simulink model "sat_sim_open_loop"  (R2022b)
settings: Solver=FixedStepAuto  StartTime=0.0  StopTime=10.0  FixedStep=0.01  RelTol=1e-3
values from neighbouring files (symbols this model uses):
  Isat = 0.00042853    [sat_params.m]
  Iwheel = 0.0019098    [sat_params.m]
  Km = -2.465    [sat_params.m]
  tau = 0.1    [sat_params.m]
libraries: slpidlib x2, simulink x1
settings Model: Creator=gigliaadmin  LastModifiedBy=micha
settings SolverCC: EnableFixedStepZeroCrossing=on

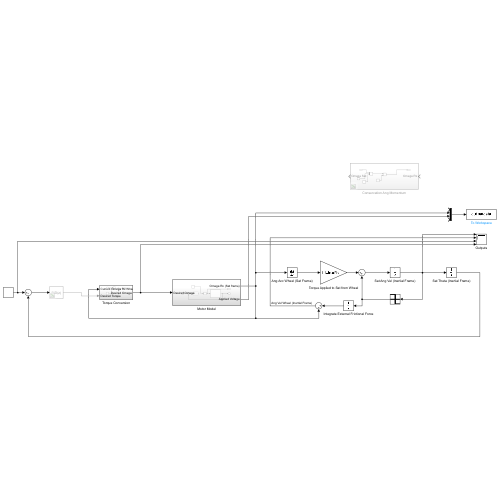
[thumbnail: Simulink's stored preview of the top-level diagram]
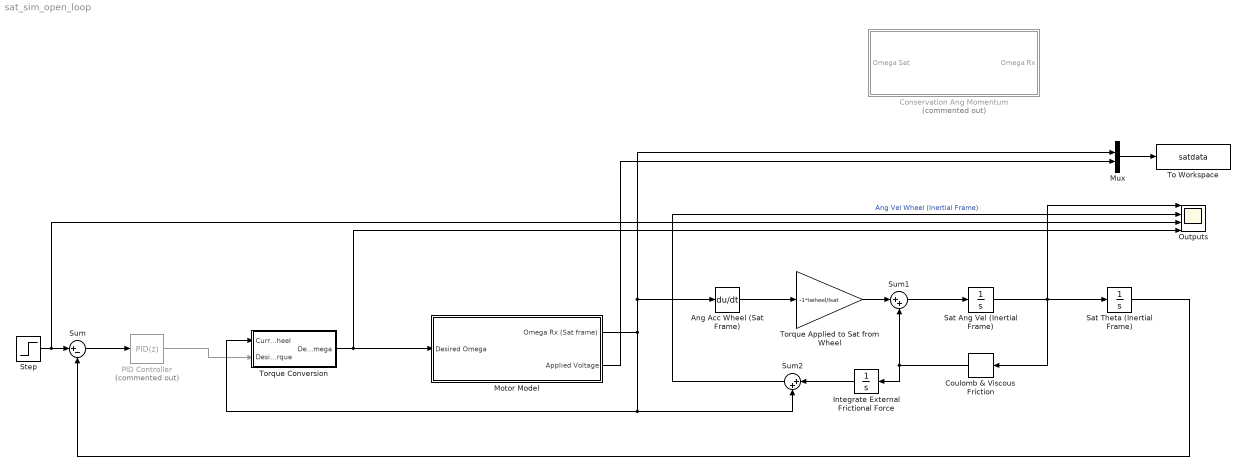
== system sat_sim_open_loop ==
  Ang Acc Wheel (Sat Frame) : Derivative
  Conservation Ang Momentum : Subsystem  Commented=on
  Coulomb & Viscous Friction : simulink/Discontinuities/Coulomb & Viscous Friction  offset=-400  gain=0
  Integrate External Frictional Force : Integrator
  Motor Model : Subsystem
  Mux : Mux
  Outputs : Scope  NumInputPorts=4
  PID Controller : slpidlib/PID Controller  Commented=on  Controller=PID  Form=Parallel  TimeDomain=Discrete-time  UseExternalTs=off  SampleTime=0.01  IntegratorMethod=Forward Euler  FilterMethod=Forward Euler  ControllerParametersSource=internal  P=8.34508860854123e-06  I=8.13072105271962e-07  UseKiTs=off  D=1.68515603832932e-05  N=100  UseFilter=off  TunerSelectOption=Transfer Function Based (PID Tuner App)  InitialConditionSource=internal  InitialConditionForIntegrator=0  InitialConditionForFilter=0  DifferentiatorICPrevScaledInput=0  ExternalReset=none  TrackingMode=off  Kt=1  LimitOutput=off  SatLimitsSource=internal  UpperSaturationLimit=inf  LowerSaturationLimit=-inf  LinearizeAsGain=on  AntiWindupMode=none  Kb=1  LimitIntegrator=off  UpperIntegratorSaturationLimit=inf  LowerIntegratorSaturationLimit=-inf  POutMin=[]  POutMax=[]  IOutMin=[]  IOutMax=[]  DOutMin=[]  DOutMax=[]  NOutMin=[]  NOutMax=[]  SumOutMin=[]  SumOutMax=[]  SaturationOutMin=[]  SaturationOutMax=[]  PParamMin=[]  PParamMax=[]  IParamMin=[]  IParamMax=[]  DParamMin=[]  DParamMax=[]  NParamMin=[]  NParamMax=[]  KbParamMin=[]  KbParamMax=[]  KtParamMin=[]  KtParamMax=[]  KbOutMin=[]  KbOutMax=[]  KtOutMin=[]  KtOutMax=[]  IntegratorOutMin=[]  IntegratorOutMax=[]  FilterOutMin=[]  FilterOutMax=[]  SumI1OutMin=[]  SumI1OutMax=[]  SumI2OutMin=[]  SumI2OutMax=[]  SumI3OutMin=[]  SumI3OutMax=[]  SumI4OutMin=[]  SumI4OutMax=[]  SumDOutMin=[]  SumDOutMax=[]  DifferentiatorOutMin=[]  DifferentiatorOutMax=[]  FilterDiffOutCoefMin=[]  FilterDiffOutCoefMax=[]  ReciprocalOutMin=[]  ReciprocalOutMax=[]  SumDenOutMin=[]  SumDenOutMax=[]  SumNumOutMin=[]  SumNumOutMax=[]  DivideOutMin=[]  DivideOutMax=[]  UdiffTsProdOutMin=[]  UdiffTsProdOutMax=[]  NTsProdOutMin=[]  NTsProdOutMax=[]  UintegralTsProdOutMin=[]  UintegralTsProdOutMax=[]  UngainTsProdOutMin=[]  UngainTsProdOutMax=[]  ClampingZeroOutDataTypeStr=Inherit: Inherit via back propagation  ClampingZeroOutMin=[]  ClampingZeroOutMax=[]  FilterDenConstantOutDataTypeStr=Inherit: Inherit via back propagation  FilterDenConstantOutMin=[]  FilterDenConstantOutMax=[]  PCopyOutDataTypeStr=Inherit: Inherit via back propagation  PCopyOutMin=[]  PCopyOutMax=[]  NCopyOutDataTypeStr=Inherit: Inherit via back propagation  NCopyOutMin=[]  NCopyOutMax=[]  IntegratorContinuousStateAttributes=''  IntegratorStateMustResolveToSignalObject=off  IntegratorRTWStateStorageClass=Auto  FilterContinuousStateAttributes=''  FilterStateMustResolveToSignalObject=off  FilterRTWStateStorageClass=Auto  ParallelPVariant=InternalParameters  IdealPVariant=Disabled  IVariant=InternalParameters  DVariant=InternalParameters  IntegratorVariant=Discrete  SatVariant=Disabled  AWVariant=Passthrough  PCopyVariant=Disabled  TRVariant=Disabled  FdbkBlocksVariant=Forward  IdealPFdbkVariant=Disabled  SatFdbkVariant=Disabled  DerivativeFilterVariant=Differentiator  NVariant=Passthrough  NCopyVariant=Disabled_SignalSpec  FilterICVariant=InternalICsDifferentiator  IntegratorICVariant=InternalICs  ExternalResetVariant=Disabled  TRSumVariant=Passthrough  SumFdbkVariant=Disabled  SumVariant=Sum_PID  TsampFilterVariant=InternalTs  TsampNgainVariant=Passthrough  TsampIntegralVariant=Passthrough  ExternalSaturationOutDataTypeStr=Inherit: Same as second input
  Sat Ang Vel (Inertial Frame) : Integrator
  Sat Theta (Inertial Frame) : Integrator
  Step : Step  After=pi  SampleTime=0
  Sum : Sum  Inputs=|+-
  Sum1 : Sum  Inputs=|++
  Sum2 : Sum  Inputs=|++
  To Workspace : ToWorkspace  VariableName=satdata  SaveFormat=Structure With Time  SampleTime=-1
  Torque Applied to Sat from Wheel : Gain  Gain=-1*Iwheel/Isat
  Torque Conversion : Subsystem
  wires:
  Sum/1 -> PID Controller/1
  PID Controller/1 -> Torque Conversion/2(Desired Torque)
  Step/1 -> Sum/1, Outputs/3
  Torque Conversion/1(Desired Omega) -> Motor Model/1(Desired Omega), Outputs/4
  Mux/1 -> To Workspace/1
  Motor Model/2(Applied Voltage) -> Mux/3
  Ang Acc Wheel (Sat Frame)/1 -> Torque Applied to Sat from Wheel/1
  Torque Applied to Sat from Wheel/1 -> Sum1/1
  Sum1/1 -> Sat Ang Vel (Inertial Frame)/1
  Sat Ang Vel (Inertial Frame)/1 -> Outputs/1, Sat Theta (Inertial Frame)/1, Coulomb & Viscous Friction/1
  Coulomb & Viscous Friction/1 -> Sum1/2, Integrate External Frictional Force/1
  Sat Theta (Inertial Frame)/1 -> Sum/2
  Motor Model/1(Omega Rx (Sat frame)) -> Ang Acc Wheel (Sat Frame)/1, Mux/2, Sum2/2, Torque Conversion/1(Current Omega Rx Wheel)
  Integrate External Frictional Force/1 -> Sum2/1
  Sum2/1 -> Outputs/2  "Ang Vel Wheel (Inertial Frame)"

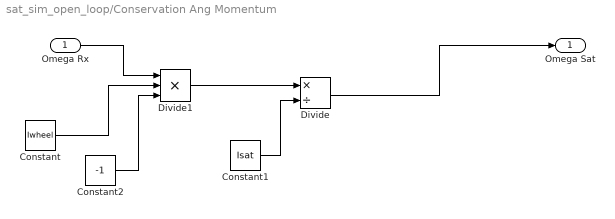
== system sat_sim_open_loop/Conservation Ang Momentum ==
  Omega Rx : Inport
  Constant : Constant  Value=Iwheel
  Constant1 : Constant  Value=Isat
  Constant2 : Constant  Value=-1
  Divide : Product  Inputs=*/
  Divide1 : Product  Inputs=***
  Omega Sat : Outport
  wires:
  Omega Rx/1 -> Divide1/1
  Constant/1 -> Divide1/2
  Divide1/1 -> Divide/1
  Constant1/1 -> Divide/2
  Divide/1 -> Omega Sat/1
  Constant2/1 -> Divide1/3

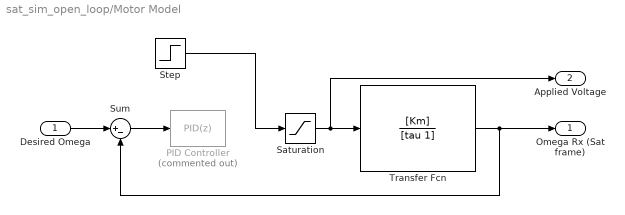
== system sat_sim_open_loop/Motor Model ==
  Desired Omega : Inport
  PID Controller : slpidlib/PID Controller  Commented=on  Controller=PID  Form=Parallel  TimeDomain=Discrete-time  UseExternalTs=off  SampleTime=0.01  IntegratorMethod=Forward Euler  FilterMethod=Forward Euler  ControllerParametersSource=internal  P=0.299316810165297  I=0.277592739548298  UseKiTs=off  D=0.00529566453574459  N=68.5493518695111  UseFilter=on  TunerSelectOption=Transfer Function Based (PID Tuner App)  InitialConditionSource=internal  InitialConditionForIntegrator=0  InitialConditionForFilter=0  DifferentiatorICPrevScaledInput=0  ExternalReset=none  TrackingMode=off  Kt=1  LimitOutput=off  SatLimitsSource=internal  UpperSaturationLimit=inf  LowerSaturationLimit=-inf  LinearizeAsGain=on  AntiWindupMode=none  Kb=1  LimitIntegrator=off  UpperIntegratorSaturationLimit=inf  LowerIntegratorSaturationLimit=-inf  POutMin=[]  POutMax=[]  IOutMin=[]  IOutMax=[]  DOutMin=[]  DOutMax=[]  NOutMin=[]  NOutMax=[]  SumOutMin=[]  SumOutMax=[]  SaturationOutMin=[]  SaturationOutMax=[]  PParamMin=[]  PParamMax=[]  IParamMin=[]  IParamMax=[]  DParamMin=[]  DParamMax=[]  NParamMin=[]  NParamMax=[]  KbParamMin=[]  KbParamMax=[]  KtParamMin=[]  KtParamMax=[]  KbOutMin=[]  KbOutMax=[]  KtOutMin=[]  KtOutMax=[]  IntegratorOutMin=[]  IntegratorOutMax=[]  FilterOutMin=[]  FilterOutMax=[]  SumI1OutMin=[]  SumI1OutMax=[]  SumI2OutMin=[]  SumI2OutMax=[]  SumI3OutMin=[]  SumI3OutMax=[]  SumI4OutMin=[]  SumI4OutMax=[]  SumDOutMin=[]  SumDOutMax=[]  DifferentiatorOutMin=[]  DifferentiatorOutMax=[]  FilterDiffOutCoefMin=[]  FilterDiffOutCoefMax=[]  ReciprocalOutMin=[]  ReciprocalOutMax=[]  SumDenOutMin=[]  SumDenOutMax=[]  SumNumOutMin=[]  SumNumOutMax=[]  DivideOutMin=[]  DivideOutMax=[]  UdiffTsProdOutMin=[]  UdiffTsProdOutMax=[]  NTsProdOutMin=[]  NTsProdOutMax=[]  UintegralTsProdOutMin=[]  UintegralTsProdOutMax=[]  UngainTsProdOutMin=[]  UngainTsProdOutMax=[]  ClampingZeroOutDataTypeStr=Inherit: Inherit via back propagation  ClampingZeroOutMin=[]  ClampingZeroOutMax=[]  FilterDenConstantOutDataTypeStr=Inherit: Inherit via back propagation  FilterDenConstantOutMin=[]  FilterDenConstantOutMax=[]  PCopyOutDataTypeStr=Inherit: Inherit via back propagation  PCopyOutMin=[]  PCopyOutMax=[]  NCopyOutDataTypeStr=Inherit: Inherit via back propagation  NCopyOutMin=[]  NCopyOutMax=[]  IntegratorContinuousStateAttributes=''  IntegratorStateMustResolveToSignalObject=off  IntegratorRTWStateStorageClass=Auto  FilterContinuousStateAttributes=''  FilterStateMustResolveToSignalObject=off  FilterRTWStateStorageClass=Auto  ParallelPVariant=InternalParameters  IdealPVariant=Disabled  IVariant=InternalParameters  DVariant=InternalParameters  IntegratorVariant=Discrete  SatVariant=Disabled  AWVariant=Passthrough  PCopyVariant=Disabled  TRVariant=Disabled  FdbkBlocksVariant=Forward  IdealPFdbkVariant=Disabled  SatFdbkVariant=Disabled  DerivativeFilterVariant=ForwardEulerFilter  NVariant=InternalParameters  NCopyVariant=Disabled  FilterICVariant=InternalICsFilter  IntegratorICVariant=InternalICs  ExternalResetVariant=Disabled  TRSumVariant=Passthrough  SumFdbkVariant=Disabled  SumVariant=Sum_PID  TsampFilterVariant=InternalTs  TsampNgainVariant=Passthrough  TsampIntegralVariant=Passthrough  ExternalSaturationOutDataTypeStr=Inherit: Same as second input
  Saturation : Saturate  UpperLimit=12  LowerLimit=-12
  Step : Step  After=12  SampleTime=0
  Sum : Sum  Inputs=|+-
  Transfer Fcn : TransferFcn  Numerator=[Km]  Denominator=[tau 1]
  Omega Rx (Sat frame) : Outport
  Applied Voltage : Outport  Port=2
  wires:
  Desired Omega/1 -> Sum/1
  Transfer Fcn/1 -> Sum/2, Omega Rx (Sat frame)/1
  Sum/1 -> PID Controller/1
  Saturation/1 -> Applied Voltage/1, Transfer Fcn/1
  Step/1 -> Saturation/1

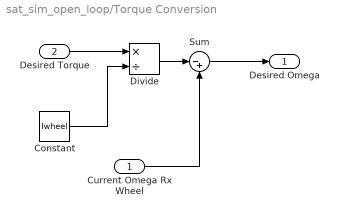
== system sat_sim_open_loop/Torque Conversion ==
  Current Omega Rx Wheel : Inport
  Desired Torque : Inport  Port=2
  Constant : Constant  Value=Iwheel
  Divide : Product  Inputs=*/
  Sum : Sum  Inputs=|-+
  Desired Omega : Outport
  wires:
  Desired Torque/1 -> Divide/1
  Constant/1 -> Divide/2
  Divide/1 -> Sum/1
  Current Omega Rx Wheel/1 -> Sum/2
  Sum/1 -> Desired Omega/1
